simulink model "first"  (R2023a)
settings: Solver=FixedStepAuto  StartTime=0.0  StopTime=1  FixedStep=0.001  RelTol=1e-3
settings Model: Creator=evdokiiagalkina  LastModifiedBy=evdokiiagalkina

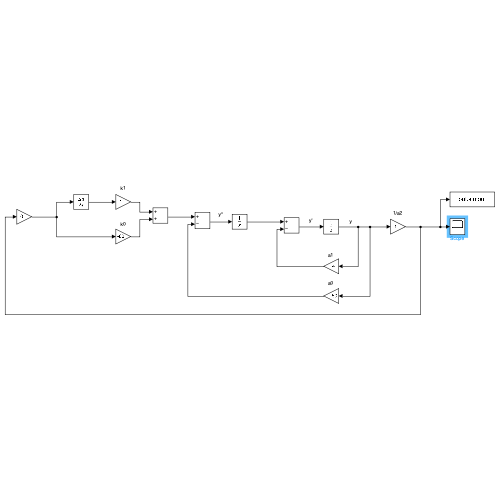
[thumbnail: Simulink's stored preview of the top-level diagram]
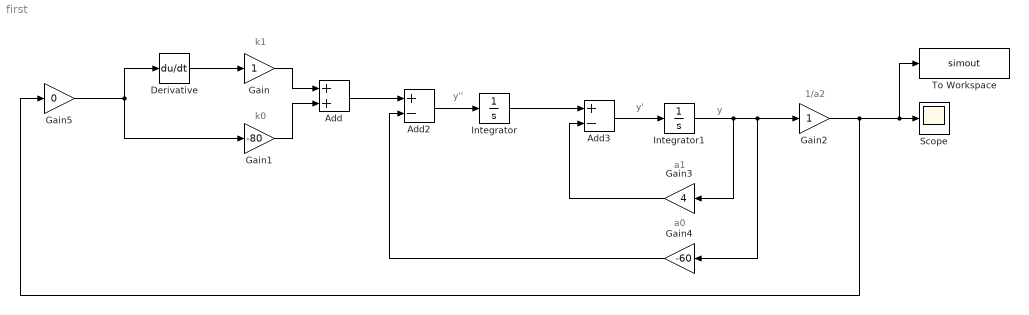
== system first ==
  note: y
  note: y'
  note: y''
  note: a1
  note: a0
  note: 1/a2
  note: k0
  note: k1
  Add : Sum
  Add2 : Sum  Inputs=+-
  Add3 : Sum  Inputs=+-
  Derivative : Derivative
  Gain : Gain
  Gain1 : Gain  Gain=-80
  Gain2 : Gain
  Gain3 : Gain  Gain=4
  Gain4 : Gain  Gain=-60
  Gain5 : Gain  Gain=0
  Integrator : Integrator  InitialCondition=5
  Integrator1 : Integrator  InitialCondition=5
  Scope : Scope
  To Workspace : ToWorkspace  VariableName=simout  SaveFormat=Timeseries  SampleTime=-1
  wires:
  Derivative/1 -> Gain/1
  Gain/1 -> Add/1
  Gain1/1 -> Add/2
  Gain5/1 -> Gain1/1, Derivative/1
  Add/1 -> Add2/1
  Add2/1 -> Integrator/1
  Integrator/1 -> Add3/1
  Add3/1 -> Integrator1/1
  Gain2/1 -> Gain5/1, Scope/1, To Workspace/1
  Integrator1/1 -> Gain3/1, Gain4/1, Gain2/1
  Gain3/1 -> Add3/2
  Gain4/1 -> Add2/2
